simulink library "vmc"  (R2021b)
settings: Solver=VariableStepAuto  StartTime=0.0  StopTime=10.0  RelTol=1e-3
undefined symbols (not defined in the file or in its folder): AVMC_ACCDeltaTqIGain4OVRD_X_kph, AVMC_ACCDeltaTqIGain4OVRD_Y_mps2, AVMC_ACCDeltaTqIGain_X_kph, AVMC_ACCDeltaTqIGain_Y_mps2, AVMC_ACCDeltaTqPGain_X_kph, AVMC_ACCDeltaTqPGain_Y_kph, AVMC_ACCLongSteadyCtrl_X_kph, AVMC_ADSPosGFBDeltaTq_X_kph, AVMC_ADSPosGFBDeltaTq_Y_mps2, AVMC_AggressJerkPCT4AT_X_kph, AVMC_AggressJerkPCT_X_kph, AVMC_AggressLimitPCT4AT_X_kph, AVMC_AggressLimitPCT_X_kph, AVMC_CCLongSteadyCtrl_X_kph, AVMC_DISCDeltaTqIGain_X_kph, AVMC_DISCDeltaTqIGain_Y_mps2, AVMC_DISCDeltaTqPGain_X_kph, AVMC_DISCDeltaTqPGain_Y_kph, AVMC_ESCRegenOut_X_kph, AVMC_ESCRegenOut_Y_Deg, AVMC_ESCRegenOutEnSpd_X_Deg, AVMC_ISOAccLimit_X_mps, AVMC_ISODecLimit_X_mps, AVMC_ISOJerk_X_mps, AVMC_LatESCRegenOut_X_kph, AVMC_LatESCRegenOut_Y_Deg, AVMC_LongAccDeadZone_X_kph, AVMC_LongAccFiltTsforP2_X_Gps, AVMC_MCPresBaseTq_X_bar, AVMC_MSALongSteadyCtrl_X_kph, AVMC_MSAPedalOvrd_X_kph, AVMC_MSASpdBand_X_kph, AVMC_MSATqDownEndTq_X_kph, AVMC_MSATqDownTime_X_kph, AVMC_OPDDisSlideRate_X_Deg, AVMC_OVRD2ActSR2FCMCMD_X_mps2, AVMC_PedalTqRWhlRatio_X_Nm, AVMC_PedalTqRWhlRatio_Y_gps, AVMC_PedalTqRWhlSlipGain_X_rat, AVMC_PedalTqRWhlSlipGain_Y_kph, AVMC_PedalTqRWhSTRGGain_X_deg, AVMC_PedalTqRWhSTRGGain_Y_kph, AVMC_RDCDetectTime_X_kph, AVMC_RDCDetectTime_Y_pct, AVMC_RDCEnSlideRate_X_Deg, AVMC_RearWhlTqRatio_X_Nm, AVMC_RearWhlTqRatio_Y_gps, AVMC_RearWhlTqSlipGain_X_rat, AVMC_RearWhlTqSlipGain_Y_kph, AVMC_RearWhlTqSTRGGain_X_deg, AVMC_RearWhlTqSTRGGain_Y_kph, AVMC_ReqBrkJoinDecSR_X_mps2, AVMC_SoftJerkPCT_X_kph, AVMC_SoftLimitPCT_X_kph, AVMC_StESCYaw_X_kph, AVMC_StESCYaw_Y_Deg, AVMC_StESCYawCom_X_kph, AVMC_StESCYawCom_Y_Gps, AVMC_TMSpdBaseTq_X_rpm, AVMC_VehHoldDecCtrlTime2_X_kph ... (+405)
libraries: hcu_lib x105, simulink x75, tqr x1, simulink_extras x1
(part 10 of 14)

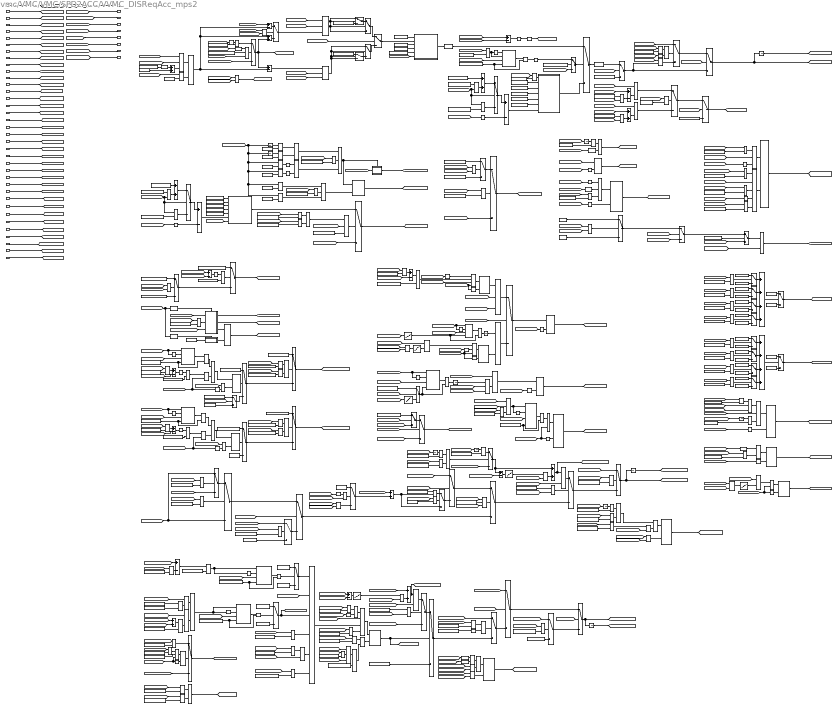
== system vmc/VMC/VMC/SPD2ACC/VVMC_DISReqAcc_mps2 ==
  note: VehHoldDelay
  note: FVT Soft Stop Control
      | (Send Hold Command after Reach H Time or ESC Standstill)
  note: Smooth Switch
      | (A, B-Pedal & REGEN to DISC)
  note: Required Acceleration for ESC
  note: Actual Required Acceleration
  note: DISC Required Acceleration
  note: Acceleration Arbitration
  note: ACC Speed Control
  note: Minimum Resolution
      | (Avoid too small command calculated from ISO Limit)
  note: Constant Speed Control
  note: ACC Constant Speed Control
  note: ACC Constant Speed Control Judgement
  VVMC_AccCalcuPID_mps2 : Inport
  VVMC_ISOJerkLimit_mps3 : Inport  Port=2
  VVMC_JerkPCT_pct : Inport  Port=3
  VVMC_ISOAccLimit_mps2 : Inport  Port=4
  VVMC_ISODecLimit_mps2 : Inport  Port=5
  VVMC_SPD2ACCAct_flg : Inport  Port=6
  VVMC_SafetyCtrl_flg : Inport  Port=7
  VINP_ACCRequiredAccel_mps2 : Inport  Port=8
  VVMC_FeatArbitrSta_enum : Inport  Port=9
  VINP_ADASACCSta_enum : Inport  Port=10
  VVMC_MeterIndSpeedForCalcu_kph : Inport  Port=11
  VVMC_FeatReqSpd_kph : Inport  Port=12
  task_time_s : Inport  Port=13
  VINP_VehSpeed_kph : Inport  Port=14
  VVMC_LongAcc_Gps : Inport  Port=15
  VVMC_LastADASWhlTqReq_Nm : Inport  Port=16
  VTQD_RrEDUAvailBrkRgnTq_Nm : Inport  Port=17
  VVMC_ACCVehHoldReqRaw_flg : Inport  Port=18
  VVMC_EstSlope_Deg : Inport  Port=19
  VTQD_FrEDUAvailBrkRgnTq_Nm : Inport  Port=20
  VVMC_ACCLowSpdTqCtrl_flg : Inport  Port=21
  VINP_GRADE_Deg : Inport  Port=22
  VINP_LFWhlRotDir_enum : Inport  Port=23
  VINP_LRWhlRotDir_enum : Inport  Port=24
  VINP_RFWhlRotDir_enum : Inport  Port=25
  VINP_RRWhlRotDir_enum : Inport  Port=26
  VVMC_ACCObjDist_m : Inport  Port=27
  VINP_MCPressure_bar : Inport  Port=28
  VDSC_PreACC_flg : Inport  Port=29
  VDSC_PreACC_mps2 : Inport  Port=30
  VDSC_DISCSta_enum : Inport  Port=31
  VDSC_AutoTurnMode_flg : Inport  Port=32
  VINP_BrkSwSta_flg : Inport  Port=33
  VINP_ACCVehHoldReq_flg : Inport  Port=34
  VTQD_GearActualPosn_enum : Inport  Port=35
  VTQD_LowIdleAccPedal_flg : Inport  Port=36
  VINP_EPBSta_enum : Inport  Port=37
  1-D Lookup Table : Lookup_n-D  NumberOfTableDimensions=1  BreakpointsForDimension1=AVMC_ReqBrkJoinDecSR_X_mps2  Table=MVMC_ReqBrkJoinDecSR_Y_mps3  InternalRulePriority=Speed  RndMeth=Simplest  InputSameDT=on
  1-D Lookup Table1 : Lookup_n-D  NumberOfTableDimensions=1  BreakpointsForDimension1=AVMC_OVRD2ActSR2FCMCMD_X_mps2  Table=MVMC_OVRD2ActSR2FCMCMD_Y_mps3  InternalRulePriority=Speed  RndMeth=Simplest  InputSameDT=on
  AND{,6,14,29} (4 alike) : Logic  Operator=OR  AllPortsSameDT=off  OutDataTypeStr=boolean
  AND{1,8,10,12,15,18..20,23..28} (14 alike) : Logic  AllPortsSameDT=off  OutDataTypeStr=boolean
  AND{3..5,11,16,21..22} (7 alike) : Logic  Inputs=3  AllPortsSameDT=off  OutDataTypeStr=boolean
  AND13 : Logic  Operator=OR  Inputs=5  AllPortsSameDT=off  OutDataTypeStr=boolean
  AND17 : Logic  Inputs=4  AllPortsSameDT=off  OutDataTypeStr=boolean
  AND2 : Logic  Inputs=4  AllPortsSameDT=off  OutDataTypeStr=boolean
  AND7 : Logic  Operator=OR  Inputs=3  AllPortsSameDT=off  OutDataTypeStr=boolean
  AND9 : Logic  Operator=OR  Inputs=3  AllPortsSameDT=off  OutDataTypeStr=boolean
  Abs{2..4,6} (4 alike) : Abs
  Add{,2,5,7,9..10,15,17..19,21,23,25} (13 alike) : Sum  Inputs=+-
  Add{1,3..4,8,11,14,16,22,24} (9 alike) : Sum
  Add12 : Sum  Inputs=++++
  Add13 : Sum  Inputs=++++
  CMDRepeat : Stateflow chart  TreatAsAtomicUnit=on
      settings: PortSchema="{\"entries\":[{\"content\":{\"sides\":[{\"content\":{\"connectorIds\":[\"In2\",\"In1\",\"In3\",\"In4\",\"In5\",\"In6\"]},\"type\":\"ConnectorPlacement.EquallySpacedRectSide\",\"uuid\":\"905b82c5-26d0-4d78-9cc9-ade9518b6cb1\"},{\"content\":{\"connectorIds\":[\"Out1\"],\"side\":\"RIGHT\"},\"type\":\"ConnectorPlacement.EquallySpacedRectSide\",\"uuid\":\"7321c4d8-dca0-41f9-ac80-faa74e816847\"},{\"content\":{\"connectorIds\":[],\"side\":\"TOP\"},\"type\":\"ConnectorPlacement.EquallySpacedRectSide\",\"uuid\":\"61a83612-f0ae-4eca-a4ee-e5180dc2049c\"}]},\"type\":\"ConnectorPlacement.EquallySpacedConnector\",\"uuid\":\"6863a8ab-8f7f-41d7-93f0-c1bbef1d5e3d\"}],\"packageUris\":[\"http://schema.mathworks.com/mf0/Connector/R2020b\"],\"version\":\"1.0\"}"
  Cast To Single : DataTypeConversion  OutDataTypeStr=single
  Cast To Single1 : DataTypeConversion  OutDataTypeStr=single
  Cast To Single7 : DataTypeConversion  OutDataTypeStr=single
  Constant : Constant  Value=pct
  Constant{1,17,27,34,38..39,42,44..45,49,64,66..68,79,81,90..92,95,108,114..115,125,127,129,131,139,141,143,145,154,163,166,175,180} (36 alike) : Constant  Value=ZERO_FLOAT
  Constant{10,94,103,107,133,147} (6 alike) : Constant  Value=TRUE
  Constant100 : Constant  Value=KVMC_VehHoldDecCtrlBSlope4ATH_mps3
  Constant101 : Constant  Value=KVMC_ReqBrkJoinWaitTime_s
  Constant{21,102,106,134,148} (5 alike) : Constant  Value=FALSE
  Constant104 : Constant  Value=KVMC_AGSVReqAccel_mps2
  Constant105 : Constant  Value=KVMC_ReqBrkJoinWaitTime_s
  Constant{7,11..12,32} (4 alike) : Constant  Value=ENUM_FEATARBITRSTA_DISC
  Constant116 : Constant  Value=KVMC_ReqBrkInDecSW_flg
  Constant{117,122..124} (4 alike) : Constant  Value=ENUM_WheelRotDir_STANDSTILL
  Constant118 : Constant  Value=KVMC_VehHoldDecCtrlBSlope_mps3
  Constant119 : Constant  Value=KVMC_VehHoldDist_m
  Constant{37,41,51,76,84,120,156,168} (8 alike) : Constant  Value=KVMC_GravityValue_mps2
  Constant{2,126,128,130,132,140,142,144,146} (9 alike) : Constant  Value=ONE_FLOAT
  Constant{6,13,33,55,61} (5 alike) : Constant  Value=ENUM_FEATARBITRSTA_ACC
  Constant{135..138} (4 alike) : Constant  Value=ENUM_WheelRotDir_BACKWARD
  Constant14 : Constant  Value=KVMC_SpdCtrlEnBand_kph
  Constant15 : Constant  Value=KVMC_VehHoldDelaySW_flg
  Constant150 : Constant  Value=KVMC_VehHoldHoldDecTime_s
  Constant151 : Constant  Value=KVMC_VehHoldDecCtrlBSlope_mps3
  Constant152 : Constant  Value=ENUM_FEATARBITRSTA_AEB
  Constant155 : Constant  Value=KVMC_VehHoldDecCtrlBSlopeCal1_mps3
  Constant157 : Constant  Value=KVMC_VehHoldHoldDecTime_s
  Constant158 : Constant  Value=KVMC_VehHoldDecCtrlBSlopeCal1_mps3
  Constant16 : Constant  Value=KVMC_Veh2MeterSpdFactor_enum
  Constant160 : Constant  Value=ENUM_VEHHOLDDELTAACCSTA_EQUAL
  Constant161 : Constant  Value=ENUM_VEHHOLDDELTAACCSTA_ACTHIGH
  Constant162 : Constant  Value=KVMC_MCPPassHoldDecTime_s
  Constant164 : Constant  Value=KVMC_VehHoldDeltaAccDB_mps2
  Constant167 : Constant  Value=KVMC_VehHoldDecCtrlBSlope_mps3
  Constant170 : Constant  Value=KVMC_VehHoldCal1BigDeltaAcc_mps2
  Constant172 : Constant  Value=KVMC_VehHoldHTimeNoMCP_bar
  Constant173 : Constant  Value=ENUM_FEATARBITRSTA_AEB
  Constant174 : Constant  Value=KVMC_VehHoldHTimeNoMCPCnt_s
  Constant176 : Constant  Value=KVMC_ReachSpeedCountTime_s
  Constant177 : Constant  Value=KVMC_ReachSpeedCount_flg
  Constant178 : Constant  Value=KVMC_DISCDecCtrlJerk_mps3
  Constant179 : Constant  Value=KVMC_DISCDecCtrlJerk_mps3
  Constant18 : Constant  Value=ENUM_ADASACCSTA_SHUTOFF
  Constant181 : Constant  Value=ENUM_DISCSTA_ACTIVE
  Constant19 : Constant  Value=ENUM_GEARACTUALPOSN_D
  Constant20 : Constant  Value=KVMC_VehHoldDecCtrlMaxDec_mps2
  Constant{22,80,85..86,99} (5 alike) : Constant  Value=ENUM_ADASACCSTA_ACTIVE
  Constant23 : Constant  Value=KVMC_Veh2MeterSpdOffset_enum
  Constant24 : Constant  Value=KVMC_SpdCtrlDisBand_kph
  Constant25 : Constant  Value=MINUSONE_FLOAT
  Constant26 : Constant  Value=KVMC_SpdCtrlReqAccel_mps2
  Constant28 : Constant  Value=KVMC_Veh2MeterSpdLoFactor_enum
  Constant29 : Constant  Value=KVMC_ADSDecShiftSW_flg
  Constant3 : Constant  Value=ZERO_INT
  Constant30 : Constant  Value=KVMC_CMDRepeatTime_enum
  Constant35 : Constant  Value=KVMC_SPD2ACCLastAccelSourceSW_flg
  Constant36 : Constant  Value=KVMC_DISCDecNoBrk_flg
  Constant4 : Constant  Value=KVMC_CMDRepeatTime_enum
  Constant40 : Constant  Value=ENUM_DISCSTA_ACTIVE
  Constant43 : Constant  Value=KVMC_AccelCtrlTqLowerLimit_Nm
  Constant46 : Constant  Value=KVMC_SprtAccelCMDSW_flg
  Constant47 : Constant  Value=KVMC_TqAccelCtrlBand_mps2
  Constant48 : Constant  Value=ENUM_EPBSTA_APPLIED
  Constant5 : Constant  Value=ENUM_FEATARBITRSTA_ACCDISC
  Constant52 : Constant  Value=KVMC_VehHoldDeltaAccDB_mps2
  Constant53 : Constant  Value=KVMC_ReqAccelLowerLimit_mps2
  Constant54 : Constant  Value=KVMC_ReqDecelLowerLimit_mps2
  Constant56 : Constant  Value=ENUM_FEATARBITRSTA_ACCDISC
  Constant57 : Constant  Value=KVMC_SpdCtrlEnBand_kph
  Constant58 : Constant  Value=KVMC_Veh2MeterSpdFactor_enum
  Constant59 : Constant  Value=KVMC_Veh2MeterSpdOffset_enum
  Constant60 : Constant  Value=KVMC_SpdCtrlDisBand_kph
  Constant62 : Constant  Value=MINUSONE_FLOAT
  Constant63 : Constant  Value=KVMC_SpdCtrlReqAccel_mps2
  Constant65 : Constant  Value=KVMC_Veh2MeterSpdLoFactor_enum
  Constant69 : Constant  Value=ENUM_VEHHOLDDELTAACCSTA_EQUAL
  Constant70 : Constant  Value=ENUM_VEHHOLDDELTAACCSTA_ACTLOW
  Constant71 : Constant  Value=KVMC_ACCSpdCtrlSW_flg
  Constant73 : Constant  Value=KVMC_ADASWhlTqLimRat_rat
  Constant74 : Constant  Value=KVMC_VehHoldDecCtrl_flg
  Constant75 : Constant  Value=KVMC_OVRD2ActRampSW_flg
  Constant77 : Constant  Value=ENUM_VEHHOLDDELTAACCSTA_EQUAL
  Constant78 : Constant  Value=ENUM_VEHHOLDDELTAACCSTA_ACTLOW
  Constant8 : Constant  Value=ENUM_FEATARBITRSTA_ACCDISC
  Constant82 : Constant  Value=KVMC_CallBrkJoinSpd_kph
  Constant83 : Constant  Value=ENUM_ADASACCSTA_OVERRIDE
  Constant87 : Constant  Value=ENUM_ADASACCSTA_OVERRIDE
  Constant88 : Constant  Value=KVMC_ADASWhlTqLimRat_rat
  Constant89 : Constant  Value=KVMC_ADSDecAlwaysShift_flg
  Constant9 : Constant  Value=KVMC_VehHoldDelayMCP_bar
  Constant93 : Constant  Value=ENUM_VEHHOLDDELTAACCSTA_ACTHIGH
  Constant96 : Constant  Value=KVMC_ADSDecRspsRatio_rat
  Constant97 : Constant  Value=KVMC_VehHoldDeltaAccDB_mps2
  ConstantSpeedControl : Stateflow chart  TreatAsAtomicUnit=on
      settings: PortSchema="{\"entries\":[{\"content\":{\"sides\":[{\"content\":{\"connectorIds\":[\"In1\",\"In3\",\"In4\",\"In5\",\"In6\",\"In7\",\"In2\"]},\"type\":\"ConnectorPlacement.EquallySpacedRectSide\",\"uuid\":\"931d4d55-b643-4b97-a7aa-1deb2b509e83\"},{\"content\":{\"connectorIds\":[\"Out1\"],\"side\":\"RIGHT\"},\"type\":\"ConnectorPlacement.EquallySpacedRectSide\",\"uuid\":\"f2f28b13-6937-4f35-b44e-683edec0d4ba\"},{\"content\":{\"connectorIds\":[],\"side\":\"TOP\"},\"type\":\"ConnectorPlacement.EquallySpacedRectSide\",\"uuid\":\"e2886b86-de2a-4a68-b05f-bfb0f2051baf\"}]},\"type\":\"ConnectorPlacement.EquallySpacedConnector\",\"uuid\":\"cece4c76-e980-42e8-adab-da09fec387c1\"}],\"packageUris\":[\"http://schema.mathworks.com/mf0/Connector/R2020b\"],\"version\":\"1.0\"}"
  ConstantSpeedControl1 : Stateflow chart  TreatAsAtomicUnit=on
      settings: PortSchema="{\"entries\":[{\"content\":{\"sides\":[{\"content\":{\"connectorIds\":[\"In2\",\"In3\",\"In4\",\"In5\",\"In6\",\"In1\",\"In7\"]},\"type\":\"ConnectorPlacement.EquallySpacedRectSide\",\"uuid\":\"931d4d55-b643-4b97-a7aa-1deb2b509e83\"},{\"content\":{\"connectorIds\":[\"Out1\"],\"side\":\"RIGHT\"},\"type\":\"ConnectorPlacement.EquallySpacedRectSide\",\"uuid\":\"f2f28b13-6937-4f35-b44e-683edec0d4ba\"},{\"content\":{\"connectorIds\":[],\"side\":\"TOP\"},\"type\":\"ConnectorPlacement.EquallySpacedRectSide\",\"uuid\":\"e2886b86-de2a-4a68-b05f-bfb0f2051baf\"}]},\"type\":\"ConnectorPlacement.EquallySpacedConnector\",\"uuid\":\"cece4c76-e980-42e8-adab-da09fec387c1\"}],\"packageUris\":[\"http://schema.mathworks.com/mf0/Connector/R2020b\"],\"version\":\"1.0\"}"
  Detect Decrease : simulink/Logic and Bit Operations/Detect Decrease  vinit=0.0  OutDataTypeStr=boolean
  Detect Increase{,1..3,5..7} (7 alike) : simulink/Logic and Bit Operations/Detect Increase  vinit=0.0  OutDataTypeStr=boolean
  Divide : Product  Inputs=*/
  Divide1 : Product  Inputs=***
  Divide{2,4..22} (20 alike) : Product  Inputs=**
  Divide24 : Product  Inputs=*/
  InitialCondition: 0 : UnitDelay  SampleTime=-1  HasFrameUpgradeWarning=on
  InitialCondition: 0 (1) : UnitDelay  SampleTime=-1  HasFrameUpgradeWarning=on
  Logical Operator2 : Logic  Operator=OR  Inputs=6  AllPortsSameDT=off  OutDataTypeStr=boolean
  Logical Operator4 : Logic  Inputs=3  AllPortsSameDT=off  OutDataTypeStr=boolean
  Logical Operator5 : Logic  Operator=OR  AllPortsSameDT=off  OutDataTypeStr=boolean
  MVMC_VehHoldDecCtrlTime2_Y : Lookup_n-D  NumberOfTableDimensions=1  BreakpointsForDimension1=AVMC_VehHoldDecCtrlTime2_X_kph  Table=MVMC_VehHoldDecCtrlTime2_Y_s  InternalRulePriority=Speed  RndMeth=Simplest  InputSameDT=on
  MVMC_VehHoldDecCtrlTime_Y_s1 : Lookup_n-D  NumberOfTableDimensions=1  BreakpointsForDimension1=AVMC_VehHoldDecCtrlTime_X_kph  Table=MVMC_VehHoldDecCtrlTime_Y_s  InternalRulePriority=Speed  RndMeth=Simplest  InputSameDT=on
  MVMC_VehHoldMCPPass2_Y_bar : Lookup_n-D  NumberOfTableDimensions=1  BreakpointsForDimension1=AVMC_VehHoldMCPPass2_X_deg  Table=MVMC_VehHoldMCPPass2_Y_bar  InternalRulePriority=Speed  RndMeth=Simplest  InputSameDT=on
  MVMC_VehHoldMCPPass_Y_bar : Lookup_n-D  NumberOfTableDimensions=1  BreakpointsForDimension1=AVMC_VehHoldMCPPass_X_deg  Table=MVMC_VehHoldMCPPass_Y_bar  InternalRulePriority=Speed  RndMeth=Simplest  InputSameDT=on
  Max1 : MinMax  Function=max  Inputs=2
  Max5 : MinMax  Function=max  Inputs=2
  Merge3 : Merge
  Min1 : MinMax  Inputs=2
  Min2 : MinMax  Function=max  Inputs=2
  Min3 : MinMax  Inputs=2
  Min4 : MinMax  Function=max  Inputs=2
  Min5 : MinMax  Inputs=2
  Min6 : MinMax  Function=max  Inputs=2
  MinMax2 : MinMax  Inputs=3
  MinMax3 : MinMax  Function=max  Inputs=3
  NOT{,1..27,29..31,33..34} (33 alike) : Logic  Operator=NOT  AllPortsSameDT=off  OutDataTypeStr=boolean
  OR{,1..4,10..15,18,20} (13 alike) : Logic  Operator=OR  AllPortsSameDT=off  OutDataTypeStr=boolean
  OR{5,16..17,21} (4 alike) : Logic  AllPortsSameDT=off  OutDataTypeStr=boolean
  OR19 : Logic  Inputs=3  AllPortsSameDT=off  OutDataTypeStr=boolean
  OR6 : Logic  Operator=OR  Inputs=3  AllPortsSameDT=off  OutDataTypeStr=boolean
  OR7 : Logic  Operator=OR  Inputs=3  AllPortsSameDT=off  OutDataTypeStr=boolean
  OR8 : Logic  Inputs=3  AllPortsSameDT=off  OutDataTypeStr=boolean
  OR9 : Logic  Operator=OR  Inputs=3  AllPortsSameDT=off  OutDataTypeStr=boolean
  Relational Operator{,1..3,5,12..14,21..23,27..28,33,43,49..56,58..59,61,69,78..79,83..86} (33 alike) : RelationalOperator  Operator===  OutDataTypeStr=boolean  RndMeth=Simplest
  Relational Operator{4,8,10,20,24..25,35,46,62} (9 alike) : RelationalOperator  Operator=<  OutDataTypeStr=boolean  RndMeth=Simplest
  Relational Operator{6,9,15..16,18,29,31,41,48,60,67..68,71,82} (14 alike) : RelationalOperator  Operator=<=  OutDataTypeStr=boolean  RndMeth=Simplest
  Relational Operator{17,19,30,32,39..40,42,57,63,65,70,72,75} (13 alike) : RelationalOperator  OutDataTypeStr=boolean  RndMeth=Simplest
  Relational Operator{26,34,36,45,47,64,66,73,76,81} (10 alike) : RelationalOperator  Operator=>  OutDataTypeStr=boolean  RndMeth=Simplest
  Relational Operator38 : RelationalOperator  Operator=~=  OutDataTypeStr=boolean  RndMeth=Simplest
  Relational Operator74 : RelationalOperator  Operator=~=  OutDataTypeStr=boolean  RndMeth=Simplest
  Relational Operator77 : RelationalOperator  Operator=~=  OutDataTypeStr=boolean  RndMeth=Simplest
  Round : Rounding  Operator=round
  Round3 : Rounding  Operator=round
  Round4 : Rounding  Operator=round
  SR_Latch{,1..17} (18 alike) : hcu_lib/Basic_Blocks/SR_Latch
  Switch : Switch  Criteria=u2 > Threshold  Threshold=KVMC_Veh2MeterSpdLoBdy_kph
  Switch1 : Switch  Criteria=u2 > Threshold  Threshold=KVMC_Veh2MeterSpdLoBdy_kph
  Switch{2..3,5..11,14,16..21,23..25,27..30,32..37,39,41..44,49} (35 alike) : Switch  Criteria=u2 > Threshold
  Switch26 : Switch  Threshold=TWO_FLOAT
  Switch31 : Switch  Threshold=TWO_FLOAT
  Timer{,1..3,5..8} (8 alike) : hcu_lib/Basic_Blocks/Timer
  Triggered Subsystem4 : Subsystem  TreatAsAtomicUnit=on
  Triggered Subsystem6 : Subsystem  TreatAsAtomicUnit=on
  Triggered Subsystem7 : Subsystem  TreatAsAtomicUnit=on
  Unit Delay{1..7,9..12} (11 alike) : UnitDelay  SampleTime=-1  HasFrameUpgradeWarning=on
  u2 > 0 (1){,1..13,15} (15 alike) : Switch  Criteria=u2 > Threshold
  u2 > 0 (10) : Switch  Criteria=u2 > Threshold
  u2 > 0 (11) : Switch  Criteria=u2 > Threshold
  u2 > 0 (16)1 : Switch  Criteria=u2 > Threshold  Threshold=KVMC_ReqAccelLowerLimit_mps2
  u2 > 0 (16)2 : Switch  Criteria=u2 > Threshold  Threshold=KVMC_ReqDecelLowerLimit_mps2
  u2 > 0 (2) : Switch  Criteria=u2 > Threshold
  u2 > 0 (5) : Switch  Criteria=u2 > Threshold
  u2 > 0 (7) : Switch  Criteria=u2 > Threshold
  u2 > 0 (9) : Switch  Criteria=u2 > Threshold
  u2 >= 0 : Switch
  "VVMC_ACCRequiredAccel_mps2 " : Outport
  VVMC_FeatArbitrFinal_enum : Outport  Port=2
  VVMC_ActACCRequiredAccel_mps2 : Outport  Port=3
  VVMC_VehHoldDecCtrlHEnd_flg : Outport  Port=4
  VVMC_DISCReqAcc_mps2 : Outport  Port=5
  VVMC_AccelTurnHold_flg : Outport  Port=6
  VVMC_ACCVehHoldReq_flg : Outport  Port=7
  VVMC_ACCShutOffHold_flg : Outport  Port=8
  VVMC_OVRD2ActRampActive_flg : Outport  Port=9
  wires:
  Switch42/1 -> InitialCondition: 0 (1)/1, [VVMC_DISCReqAcc_mps2]  "VVMC_DISCReqAcc_mps2"
  Switch2/1 -> [VVMC_JerkSource_mps2], Add/1, Add1/2  "VVMC_JerkSource_mps2"
  [VVMC_DISCReqAcc_mps2] -> u2 > 0 (9)/1, u2 > 0 (2)/3
  Relational Operator5/1 -> u2 > 0 (9)/2
  [VVMC_AfterCtrlACCReqAccel_mps2] -> u2 > 0 (9)/3
  InitialCondition: 0/1 -> [VVMC_LastActACCRequiredAccel_mps2]  "VVMC_LastActACCRequiredAccel_mps2"
  u2 > 0 (5)/1 -> u2 > 0 (1)/3
  u2 > 0 (2)/1 -> u2 > 0 (1)/1
  [VVMC_SPD2ACCAct_flg] -> u2 > 0 (1)/2
  [VVMC_FeatArbitrSta_enum] -> Relational Operator1/1
  [VVMC_FeatArbitrSta_enum] -> Relational Operator2/1
  Constant1/1 -> u2 > 0 (5)/3
  Constant11/1 -> Relational Operator5/2
  Constant5/1 -> Relational Operator1/2
  Relational Operator1/1 -> u2 > 0 (2)/2
  Constant6/1 -> Relational Operator2/2
  u2 > 0 (9)/1 -> u2 > 0 (2)/1
  Relational Operator2/1 -> u2 > 0 (5)/2
  [VVMC_AfterCtrlACCReqAccel_mps2] -> u2 > 0 (5)/1
  u2 > 0 (1)9/1 -> [VVMC_ActACCRequiredAccel_mps2], InitialCondition: 0/1  "VVMC_ActACCRequiredAccel_mps2"
  [VVMC_FeatArbitrFinal_enum] -> Relational Operator5/1
  task_time_s/1 -> [task_time_s]
  [VVMC_MeterIndSpeedForCalcu_kph] -> Add2/2
  [VVMC_FeatReqSpd_kph] -> Add2/1
  u2 > 0 (11)/1 -> Cast To Single1/1
  Abs2/1 -> Round/1
  Add2/1 -> Abs2/1
  VVMC_MeterIndSpeedForCalcu_kph/1 -> [VVMC_MeterIndSpeedForCalcu_kph]
  VVMC_FeatReqSpd_kph/1 -> [VVMC_FeatReqSpd_kph]
  Cast To Single7/1 -> u2 > 0 (11)/1  "VVMC_DISCReqAccAftRepeat_mps2"
  InitialCondition: 0 (1)/1 -> [VVMC_LastDISCReqAcc_mps2]  "VVMC_LastDISCReqAcc_mps2"
  Constant13/1 -> u2 > 0 (10)/1
  Constant12/1 -> u2 > 0 (10)/3
  Relational Operator6/1 -> u2 > 0 (10)/2
  [VVMC_AfterCtrlACCReqAccel_mps2] -> Relational Operator6/1
  [VVMC_DISCReqAcc_mps2] -> Relational Operator6/2
  VINP_ADASACCSta_enum/1 -> [VINP_ADASACCSta_enum]
  [VVMC_FeatArbitrFinal_enum] -> VVMC_FeatArbitrFinal_enum/1
  u2 > 0 (7)/1 -> [VVMC_FeatArbitrFinal_enum]  "VVMC_FeatArbitrFinal_enum"
  [VVMC_FeatArbitrSta_enum] -> u2 > 0 (7)/3
  u2 > 0 (10)/1 -> u2 > 0 (7)/1
  Relational Operator3/1 -> u2 > 0 (7)/2
  [VVMC_FeatArbitrSta_enum] -> Relational Operator3/1
  Constant8/1 -> Relational Operator3/2
  VVMC_FeatArbitrSta_enum/1 -> [VVMC_FeatArbitrSta_enum]
  VINP_ACCRequiredAccel_mps2/1 -> [VINP_ACCRequiredAccel_mps2]
  VVMC_SafetyCtrl_flg/1 -> [VVMC_SafetyCtrl_flg]
  Constant4/1 -> CMDRepeat/5(KVMC_CMDRepeatTime_enum)
  Constant3/1 -> CMDRepeat/4(ZERO_INT)
  [VVMC_ACCRequiredAccel_mps2] -> "VVMC_ACCRequiredAccel_mps2 "/1
  [VVMC_ISOJerkLimit_mps3] -> Divide1/1
  Constant/1 -> Divide/2
  VVMC_SPD2ACCAct_flg/1 -> [VVMC_SPD2ACCAct_flg]
  VVMC_ISODecLimit_mps2/1 -> [VVMC_ISODecLimit_mps2]
  VVMC_ISOAccLimit_mps2/1 -> [VVMC_ISOAccLimit_mps2]
  VVMC_JerkPCT_pct/1 -> [VVMC_JerkPCT_pct]
  VVMC_ISOJerkLimit_mps3/1 -> [VVMC_ISOJerkLimit_mps3]
  VVMC_AccCalcuPID_mps2/1 -> [VVMC_AccCalcuPID_mps2]
  [VVMC_AccCalcuPID_mps2] -> u2 >= 0/2
  [VVMC_AccCalcuPID_mps2] -> MinMax3/3
  [VVMC_AccCalcuPID_mps2] -> MinMax2/1
  [VVMC_JerkPCT_pct] -> Divide/1
  Divide1/1 -> Divide2/1
  [VVMC_ISODecLimit_mps2] -> MinMax3/2
  Divide2/1 -> Add/2, Add23/2, Add1/1  "VVMC_ISOJerkLimitFinal_mps3"
  MinMax2/1 -> Switch49/3, Switch49/2, u2 > 0 (16)1/2, u2 > 0 (16)1/1
  [VVMC_ISOAccLimit_mps2] -> MinMax2/2
  Divide/1 -> Divide2/2
  u2 >= 0/1 -> CMDRepeat/1(VVMC_DISCReqAccAftLim_mps2)  "VVMC_DISCReqAccAftLim_mps2"
  CMDRepeat/1(VVMC_DISCReqAccAftRepeat_mps2) -> Cast To Single7/1
  Add/1 -> MinMax3/1
  VINP_VehSpeed_kph/1 -> [VINP_VehSpeed_kph]
  Divide5/1 -> Add4/2
  [VINP_VehSpeed_kph] -> Switch/2, Divide8/1, Divide5/2
  Constant23/1 -> Add4/1
  Constant16/1 -> Divide5/1
  Add4/1 -> Switch/1
  Round3/1 -> Add5/2
  Add5/1 -> ConstantSpeedControl/2(DeltaSpeed)
  Constant14/1 -> ConstantSpeedControl/3(KVMC_SpdCtrlEnBand_kph)
  Constant24/1 -> ConstantSpeedControl/4(KVMC_SpdCtrlDisBand_kph)
  Constant25/1 -> ConstantSpeedControl/5(MINUSONE_FLOAT)
  [VVMC_FeatReqSpd_kph] -> Round3/1
  Constant26/1 -> ConstantSpeedControl/6(KVMC_SpdCtrlReqAccel_mps2)
  Constant27/1 -> ConstantSpeedControl/7(ZERO_FLOAT)
  Divide8/1 -> Switch/3
  Constant28/1 -> Divide8/2
  Switch/1 -> Add5/1
  ConstantSpeedControl/1(ReqAccel) -> u2 > 0 (11)/3  "VVMC_DISCConSpdCtrlCMD_mps2"
  [VVMC_SPD2ACCAct_flg] -> Detect Increase/1
  VVMC_LongAcc_Gps/1 -> [VVMC_LongAcc_Gps]
  Constant35/1 -> Logical Operator4/2
  Detect Increase/1 -> Logical Operator4/1
  Logical Operator4/1 -> Switch2/2
  [VVMC_LastDISCReqAcc_mps2] -> Switch2/3
  [VVMC_LongAcc_Gps] -> Unit Delay1/1
  Constant37/1 -> Divide9/2
  Divide9/1 -> Switch2/1
  [VVMC_SPD2ACCAct_flg] -> Switch7/2
  Constant42/1 -> Switch7/3
  Constant49/1 -> Relational Operator19/2
  Constant45/1 -> u2 > 0 (1)1/3
  Logical Operator2/1 -> AND2/3
  [VVMC_LongAcc_Gps] -> Divide10/1
  Constant47/1 -> Relational Operator18/2
  [VVMC_ActACCRequiredAccel_mps2] -> Relational Operator19/1
  Constant44/1 -> Relational Operator17/2
  Relational Operator17/1 -> AND/1
  [VVMC_LastADASWhlTqReq_Nm] -> Relational Operator15/1
  u2 > 0 (1)1/1 -> u2 > 0 (1)3/3
  Constant46/1 -> NOT/1
  NOT/1 -> AND/2
  AND/1 -> u2 > 0 (1)3/2
  Relational Operator15/1 -> Logical Operator5/2
  [VTQD_RrEDUAvailBrkRgnTq_Nm] -> Add14/1
  Relational Operator16/1 -> Logical Operator5/1
  Constant43/1 -> Divide22/1
  [VVMC_ActACCRequiredAccel_mps2] -> Relational Operator17/1
  [VVMC_ActACCReqAcc4ADS_mps2] -> u2 > 0 (1)2/1
  [VVMC_ACCVehHoldReqRaw_flg] -> u2 > 0 (1)2/2
  Add7/1 -> Relational Operator18/1
  [VVMC_ActACCRequiredAccel_mps2] -> Add7/1
  SR_Latch3/1 -> [VVMC_ReqBrkJoin_flg], u2 > 0 (1)1/2  "VVMC_ReqBrkJoin_flg"
  u2 > 0 (1)3/1 -> u2 > 0 (1)2/3
  [VVMC_LastADASWhlTqReq_Nm] -> Relational Operator16/1
  Divide10/1 -> Add7/2
  Constant41/1 -> Divide10/2
  [VVMC_ActACCRequiredAccel_mps2] -> u2 > 0 (1)3/1
  u2 > 0 (1)4/1 -> [VVMC_ACCRequiredAccel_mps2], Unit Delay6/1
  Relational Operator13/1 -> OR/1
  Constant32/1 -> Relational Operator13/2
  Constant33/1 -> Relational Operator14/2
  OR/1 -> [VVMC_ReqAccelActive_flg]  "VVMC_ReqAccelActive_flg"
  [VVMC_FeatArbitrFinal_enum] -> Relational Operator13/1
  [VVMC_FeatArbitrFinal_enum] -> Relational Operator14/1
  Relational Operator14/1 -> OR/2
  [VVMC_ReqAccelActive_flg] -> u2 > 0 (1)4/2
  u2 > 0 (1)2/1 -> u2 > 0 (1)4/1
  Constant34/1 -> u2 > 0 (1)11/3
  [VVMC_ReqAccelActive_flg] -> AND2/2
  [VVMC_ActACCRequiredAccel_mps2] -> Relational Operator20/1
  Constant39/1 -> Relational Operator20/2
  Relational Operator20/1 -> AND2/4
  VTQD_RrEDUAvailBrkRgnTq_Nm/1 -> [VTQD_RrEDUAvailBrkRgnTq_Nm]
  VVMC_LastADASWhlTqReq_Nm/1 -> [VVMC_LastADASWhlTqReq_Nm]
  [VVMC_ActACCRequiredAccel_mps2] -> VVMC_ActACCRequiredAccel_mps2/1
  Constant53/1 -> u2 > 0 (16)1/3
  u2 > 0 (16)1/1 -> Switch49/1
  Constant54/1 -> u2 > 0 (16)2/1
  MinMax3/1 -> Switch6/2, Switch6/1, u2 > 0 (16)2/2, u2 > 0 (16)2/3
  Unit Delay1/1 -> Divide9/1
  AND1/1 -> Logical Operator2/5
  Relational Operator21/1 -> AND1/1
  [VVMC_FeatArbitrFinal_enum] -> Relational Operator21/1
  Constant61/1 -> Relational Operator21/2
  [VVMC_SafetyCtrl_flg] -> AND1/2
  Constant55/1 -> Relational Operator22/2
  [VVMC_FeatArbitrSta_enum] -> Relational Operator22/1
  Constant56/1 -> Relational Operator23/2
  [VVMC_FeatArbitrSta_enum] -> Relational Operator23/1
  Relational Operator23/1 -> OR1/1
  Relational Operator22/1 -> OR1/2
  Constant58/1 -> Divide11/1
  [VINP_VehSpeed_kph] -> Switch1/2, Divide12/1, Divide11/2
  Divide11/1 -> Add8/2
  Constant65/1 -> Divide12/2
  ConstantSpeedControl1/1(ReqAccel) -> Switch5/1  "VVMC_ACCConSpdCtrlCMD_mps2"
  Add9/1 -> ConstantSpeedControl1/1(DeltaSpeed)
  Constant63/1 -> ConstantSpeedControl1/5(KVMC_SpdCtrlReqAccel_mps2)
  Constant64/1 -> ConstantSpeedControl1/6(ZERO_FLOAT)
  [VVMC_ACCReqSpdMemory_kph] -> Round4/1
  Constant60/1 -> ConstantSpeedControl1/3(KVMC_SpdCtrlDisBand_kph)
  Switch1/1 -> Add9/1
  Divide12/1 -> Switch1/3
  Constant59/1 -> Add8/1
  Add8/1 -> Switch1/1
  Constant57/1 -> ConstantSpeedControl1/2(KVMC_SpdCtrlEnBand_kph)
  Round4/1 -> Add9/2
  Constant62/1 -> ConstantSpeedControl1/4(MINUSONE_FLOAT)
  Unit Delay2/1 -> Relational Operator24/1
  Constant66/1 -> Relational Operator24/2
  OR5/1 -> AND3/3
  Relational Operator24/1 -> OR4/1
  AND3/1 -> SR_Latch4/1, Triggered Subsystem4/Trigger
  Triggered Subsystem4/1(Out1) -> [VVMC_ACCReqSpdMemory_kph]  "VVMC_ACCReqSpdMemory_kph"
  SR_Latch4/1 -> [VVMC_ACCSpdCtrl_flg]  "VVMC_ACCSpdCtrl_flg"
  OR1/1 -> AND4/1
  [VVMC_ACCSpdCtrl_flg] -> AND4/2
  Constant71/1 -> AND4/3
  AND4/1 -> Switch5/2
  [VINP_ACCRequiredAccel_mps2] -> Switch5/3
  Switch5/1 -> [VVMC_AfterCtrlACCReqAccel_mps2]  "VVMC_AfterCtrlACCReqAccel_mps2"
  VVMC_ACCVehHoldReqRaw_flg/1 -> [VVMC_ACCVehHoldReqRaw_flg]
  [VVMC_ACCVehHoldReqRaw_flg] -> AND5/1
  Constant74/1 -> AND5/2
  AND5/1 -> u2 > 0 (1)5/2
  VVMC_EstSlope_Deg/1 -> [VVMC_EstSlope_Deg]
  [VVMC_ACCVehHoldReqRaw_flg] -> Detect Decrease/1, Detect Increase2/1
  Detect Increase2/1 -> Triggered Subsystem6/Trigger
  [VVMC_LastActACCRequiredAccel_mps2] -> Triggered Subsystem6/3(In3)
  Merge3/1 -> [VVMC_VehHoldEnReqAccel_mps2]  "VVMC_VehHoldEnReqAccel_mps2"
  Constant79/1 -> Triggered Subsystem7/1(In1)
  Detect Decrease/1 -> Triggered Subsystem7/Trigger
  Triggered Subsystem6/3(Out3) -> Merge3/1
  Triggered Subsystem7/1(Out1) -> Merge3/2
  Switch33/1 -> [VVMC_VehHoldDecCtrlBSlope_mps3]  "VVMC_VehHoldDecCtrlBSlope_mps3"
  [VVMC_LastActACCRequiredAccel_mps2] -> Add11/1
  Switch9/1 -> Add11/2
  [VVMC_ACCVehHoldReqRaw_flg] -> NOT1/1, Timer/1
  NOT1/1 -> Timer/2
  [task_time_s] -> Timer/3
  MVMC_VehHoldDecCtrlTime_Y_s1/1 -> Relational Operator30/2, Timer/4
  Timer/1 -> Relational Operator30/1
  Constant81/1 -> Switch9/1
  [task_time_s] -> Divide16/2
  [VVMC_VehHoldDecCtrlBSlope_mps3] -> Divide16/1
  Divide16/1 -> Switch9/3
  [VVMC_VehHoldDecCtrlBEnd_flg] -> OR3/2
  [VVMC_ACCVehHoldReqRaw_flg] -> NOT2/1
  NOT2/1 -> OR3/1
  OR3/1 -> Switch9/2
  [VVMC_VehHoldDecCtrlBEnd_flg] -> NOT3/1, Timer1/1
  [task_time_s] -> Timer1/3
  MVMC_VehHoldDecCtrlTime2_Y/1 -> Switch21/3
  Timer1/1 -> Relational Operator32/1
  SR_Latch12/1 -> [VVMC_VehHoldDecCtrlHEnd_flg]  "VVMC_VehHoldDecCtrlHEnd_flg"
  Add11/1 -> Min1/2, Switch8/3
  [VVMC_VehHoldDecCtrlHEnd_flg] -> u2 > 0 (1)6/2
  u2 > 0 (1)6/1 -> u2 > 0 (1)5/1  "VVMC_VehHoldDecCtrlAccel_mps2"
  [VVMC_VehHoldDecCtrlHEnd_flg] -> VVMC_VehHoldDecCtrlHEnd_flg/1
  Relational Operator30/1 -> Unit Delay3/1
  [VVMC_ACCVehHoldReqRaw_flg] -> AND8/1
  Relational Operator32/1 -> Unit Delay4/1
  Unit Delay4/1 -> AND7/1
  Constant90/1 -> Relational Operator34/2
  Unit Delay5/1 -> Relational Operator34/1
  Relational Operator34/1 -> OR4/2
  Constant92/1 -> Relational Operator36/2
  Constant91/1 -> Relational Operator35/2
  Relational Operator36/1 -> NOT4/1
  NOT4/1 -> OR5/2
  Relational Operator35/1 -> NOT5/1
  NOT5/1 -> OR5/1
  OR4/1 -> AND3/1
  Constant67/1 -> Relational Operator25/2
  Constant68/1 -> Relational Operator26/2
  [VINP_ACCRequiredAccel_mps2] -> Unit Delay2/1, Relational Operator36/1, Relational Operator26/1, Relational Operator25/1, Relational Operator35/1, Unit Delay5/1
  Relational Operator25/1 -> OR6/1
  Relational Operator26/1 -> OR6/3
  AND7/1 -> AND8/2
  VTQD_FrEDUAvailBrkRgnTq_Nm/1 -> [VTQD_FrEDUAvailBrkRgnTq_Nm]
  [VTQD_FrEDUAvailBrkRgnTq_Nm] -> Add14/2
  NOT3/1 -> Timer1/2
  VVMC_ACCLowSpdTqCtrl_flg/1 -> [VVMC_ACCLowSpdTqCtrl_flg]
  [VVMC_ACCLowSpdTqCtrl_flg] -> Logical Operator2/2
  [VINP_VehSpeed_kph] -> Relational Operator31/1
  Constant82/1 -> Relational Operator31/2
  Relational Operator31/1 -> Logical Operator2/4
  [VVMC_SPD2ACCAct_flg] -> CMDRepeat/6(VVMC_SPD2ACCAct_flg)
  Constant94/1 -> CMDRepeat/2(TRUE)
  Constant95/1 -> CMDRepeat/3(ZERO_FLOAT)
  [VVMC_MeterIndSpeedForCalcu_kph] -> Triggered Subsystem4/1(In1)
  Relational Operator38/1 -> OR6/2
  Constant101/1 -> Relational Operator40/2, Timer2/4
  [task_time_s] -> Timer2/3
  Logical Operator5/1 -> Timer2/1, NOT6/1
  NOT6/1 -> Timer2/2
  Timer2/1 -> Relational Operator40/1
  Relational Operator40/1 -> u2 > 0 (1)7/2
  Constant102/1 -> u2 > 0 (1)7/3
  u2 > 0 (1)7/1 -> [VVMC_ADASWhlTqReachLim_flg], Logical Operator2/3  "VVMC_ADASWhlTqReachLim_flg"
  Constant103/1 -> u2 > 0 (1)7/1
  [VVMC_ActACCRequiredAccel_mps2] -> Relational Operator41/1
  Relational Operator41/1 -> Logical Operator2/6
  Constant104/1 -> Relational Operator41/2
  Constant107/1 -> u2 > 0 (1)8/1
  Constant106/1 -> u2 > 0 (1)8/3
  Relational Operator42/1 -> u2 > 0 (1)8/2
  Timer3/1 -> Relational Operator42/1
  NOT7/1 -> Timer3/2
  Relational Operator18/1 -> NOT7/1, Timer3/1
  [task_time_s] -> Timer3/3
  Constant105/1 -> Timer3/4, Relational Operator42/2
  u2 > 0 (1)8/1 -> Logical Operator2/1
  [VINP_VehSpeed_kph] -> Triggered Subsystem6/1(In1)
  Triggered Subsystem6/1(Out1) -> [VVMC_VehHoldEnSpd_kph]  "VVMC_VehHoldEnSpd_kph"
  [VVMC_LastActACCRequiredAccel_mps2] -> u2 > 0 (1)6/1
  [VVMC_VehHoldEnSpd_kph] -> MVMC_VehHoldDecCtrlTime_Y_s1/1
  [VVMC_VehHoldEnSpd_kph] -> MVMC_VehHoldDecCtrlTime2_Y/1
  [VVMC_ACCVehHoldReqRaw_flg] -> OR8/2
  [VVMC_ACCVehHoldReqRaw_flg] -> NOT8/1
  SR_Latch5/1 -> [VVMC_ZeroSpdHoldAllow_flg]  "VVMC_ZeroSpdHoldAllow_flg"
  [VVMC_ZeroSpdHoldAllow_flg] -> AND7/2
  VINP_GRADE_Deg/1 -> [VINP_GRADE_Deg]
  OR8/1 -> SR_Latch5/1
  VINP_LFWhlRotDir_enum/1 -> [VINP_LFWhlRotDir_enum]
  VINP_LRWhlRotDir_enum/1 -> [VINP_LRWhlRotDir_enum]
  VINP_RFWhlRotDir_enum/1 -> [VINP_RFWhlRotDir_enum]
  VINP_RRWhlRotDir_enum/1 -> [VINP_RRWhlRotDir_enum]
  [VINP_LFWhlRotDir_enum] -> Relational Operator49/1
  Constant117/1 -> Relational Operator49/2
  Constant122/1 -> Relational Operator50/2
  [VINP_LRWhlRotDir_enum] -> Relational Operator50/1
  Constant123/1 -> Relational Operator51/2
  [VINP_RFWhlRotDir_enum] -> Relational Operator51/1
  [VINP_RRWhlRotDir_enum] -> Relational Operator52/1
  Constant124/1 -> Relational Operator52/2
  Relational Operator49/1 -> Switch14/2
  Constant125/1 -> Switch14/3
  Constant126/1 -> Switch14/1
  Constant128/1 -> Switch23/1
  Constant127/1 -> Switch23/3
  Relational Operator50/1 -> Switch23/2
  Relational Operator51/1 -> Switch24/2
  Constant129/1 -> Switch24/3
  Constant130/1 -> Switch24/1
  Constant132/1 -> Switch25/1
  Constant131/1 -> Switch25/3
  Relational Operator52/1 -> Switch25/2
  Switch25/1 -> Add12/4
  Switch24/1 -> Add12/3
  Switch23/1 -> Add12/2
  Switch14/1 -> Add12/1
  Add12/1 -> Switch26/2
  Constant133/1 -> Switch26/1
  Constant134/1 -> Switch26/3
  Switch26/1 -> [VVMC_WhlStandstill_flg]  "VVMC_WhlStandstill_flg"
  Switch31/1 -> [VVMC_WhlBackward_flg]  "VVMC_WhlBackward_flg"
  Constant148/1 -> Switch31/3
  Constant147/1 -> Switch31/1
  Add13/1 -> Switch31/2
  Switch27/1 -> Add13/1
  Switch28/1 -> Add13/2
  Switch29/1 -> Add13/3
  Switch30/1 -> Add13/4
  Relational Operator56/1 -> Switch30/2
  Constant145/1 -> Switch30/3
  Constant146/1 -> Switch30/1
  Constant144/1 -> Switch29/1
  Constant143/1 -> Switch29/3
  Relational Operator55/1 -> Switch29/2
  Relational Operator54/1 -> Switch28/2
  Constant141/1 -> Switch28/3
  Constant142/1 -> Switch28/1
  Constant140/1 -> Switch27/1
  Constant139/1 -> Switch27/3
  Relational Operator53/1 -> Switch27/2
  Constant138/1 -> Relational Operator56/2
  [VINP_RRWhlRotDir_enum] -> Relational Operator56/1
  [VINP_RFWhlRotDir_enum] -> Relational Operator55/1
  Constant137/1 -> Relational Operator55/2
  [VINP_LRWhlRotDir_enum] -> Relational Operator54/1
  Constant136/1 -> Relational Operator54/2
  Constant135/1 -> Relational Operator53/2
  [VINP_LFWhlRotDir_enum] -> Relational Operator53/1
  OR7/1 -> OR8/1
  [VVMC_WhlStandstill_flg] -> OR7/2
  [VVMC_WhlBackward_flg] -> OR7/3
  VVMC_ACCObjDist_m/1 -> [VVMC_ACCObjDist_m]
  [VVMC_ACCObjDist_m] -> Relational Operator48/1
  Relational Operator48/1 -> OR7/1
  Constant119/1 -> Relational Operator48/2
  [VVMC_VehHoldDecCtrlBSlopeCal1_mps3] -> Switch33/3
  Switch18/1 -> Switch33/1
  Relational Operator57/1 -> AND15/1
  VINP_MCPressure_bar/1 -> [VINP_MCPressure_bar]
  [VINP_MCPressure_bar] -> Relational Operator57/1
  SR_Latch2/1 -> [VVMC_VehHoldMCPPass_flg]  "VVMC_VehHoldMCPPass_flg"
  [VINP_GRADE_Deg] -> Max5/1
  [VVMC_EstSlope_Deg] -> Max5/2
  Max5/1 -> MVMC_VehHoldMCPPass_Y_bar/1
  MVMC_VehHoldMCPPass_Y_bar/1 -> Relational Operator57/2
  [VVMC_VehHoldDecCtrlCalSW2_flg] -> Switch33/2
  AND18/1 -> SR_Latch1/1
  Detect Increase5/1 -> AND18/1
  [VVMC_ACCVehHoldReqRaw_flg] -> NOT12/1
  [VVMC_ACCVehHoldReqRaw_flg] -> Detect Increase5/1
  SR_Latch1/1 -> [VVMC_VehHoldDecCtrlCalSW2_flg]  "VVMC_VehHoldDecCtrlCalSW2_flg"
  [VVMC_ACCVehHoldReqRaw_flg] -> AND15/2, NOT10/1
  Constant152/1 -> Relational Operator59/2
  [VVMC_FeatArbitrSta_enum] -> Relational Operator59/1
  Relational Operator59/1 -> u2 > 0 (1)9/2
  [VINP_ACCRequiredAccel_mps2] -> u2 > 0 (1)9/1
  [VVMC_VehHoldDecCtrlCalSW2_flg] -> Switch21/2
  Switch21/1 -> Relational Operator32/2, Timer1/4
  Constant162/1 -> Switch21/1
  [VVMC_ActACCRequiredAccel_mps2] -> Unit Delay9/1
  Relational Operator62/1 -> OR8/3
  Constant163/1 -> Relational Operator62/2
  Unit Delay9/1 -> Relational Operator62/1
  Constant86/1 -> Relational Operator33/2
  [VINP_ADASACCSta_enum] -> Relational Operator33/1
  Relational Operator33/1 -> AND3/2
  [VINP_ADASACCSta_enum] -> Relational Operator38/1
  Constant99/1 -> Relational Operator38/2
  [VVMC_AccelTurnHold_flg] -> Switch18/2
  [VVMC_VehHoldDecCtrlBSlopeCal2_mps3] -> Switch18/3
  Constant100/1 -> Switch18/1
  [VVMC_HoldDelayAllow_flg] -> AND5/3
  [VVMC_DISCReqAcc_mps2] -> VVMC_DISCReqAcc_mps2/1
  [VVMC_ACCSpdCtrl_flg] -> NOT13/1
  NOT13/1 -> AND6/2
  [VINP_MCPressure_bar] -> Relational Operator4/1
  Constant9/1 -> Relational Operator4/2
  Relational Operator4/1 -> AND18/2
  Constant20/1 -> Min1/1
  [VINP_MCPressure_bar] -> Relational Operator8/1
  MVMC_VehHoldMCPPass2_Y_bar/1 -> Relational Operator8/2
  Relational Operator8/1 -> AND16/1
  [VVMC_ACCVehHoldReqRaw_flg] -> AND16/3, NOT17/1
  AND16/1 -> SR_Latch/1
  NOT17/1 -> SR_Latch/2
  [VVMC_VehHoldDecCtrlCalSW2_flg] -> NOT18/1
  NOT18/1 -> AND16/2
  Min1/1 -> Switch8/1
  Max1/1 -> MVMC_VehHoldMCPPass2_Y_bar/1
  [VVMC_EstSlope_Deg] -> Max1/2
  [VINP_GRADE_Deg] -> Max1/1
  [VVMC_LastACCRequiredAccel_mps2] -> Add3/1
  1-D Lookup Table/1 -> Divide15/1
  [task_time_s] -> Divide15/2
  Divide15/1 -> Add3/2
  Min2/1 -> u2 > 0 (1)10/1
  Add3/1 -> [VVMC_ACCReqAccelAfterSR_mps2], Min2/1
  u2 > 0 (1)10/1 -> u2 > 0 (1)1/1
  Constant116/1 -> AND20/1
  [VVMC_ActACCReqAcc4ADS_mps2] -> u2 > 0 (1)10/3
  NOT8/1 -> SR_Latch5/2
  NOT12/1 -> SR_Latch1/2
  NOT10/1 -> SR_Latch2/2
  AND15/1 -> SR_Latch2/1
  Relational Operator19/1 -> OR18/1
  AND2/1 -> SR_Latch3/1
  OR6/1 -> SR_Latch4/2
  [VVMC_LongAcc_Gps] -> Divide17/1
  Triggered Subsystem6/2(Out2) -> [VVMC_VehHoldEnActAccel_mps2]  "VVMC_VehHoldEnActAccel_mps2"
  Constant51/1 -> Divide17/2
  Divide17/1 -> Triggered Subsystem6/2(In2)
  [VVMC_VehHoldEnActAccel_mps2] -> Add15/1
  [VVMC_VehHoldEnReqAccel_mps2] -> Add15/2
  Add15/1 -> Abs6/1
  Abs6/1 -> Relational Operator9/1
  Constant52/1 -> Relational Operator9/2
  Relational Operator9/1 -> Switch20/2
  [VVMC_VehHoldEnActAccel_mps2] -> Relational Operator10/1
  [VVMC_VehHoldEnReqAccel_mps2] -> Relational Operator10/2
  Switch32/1 -> Switch20/3
  Relational Operator10/1 -> Switch32/2
  Constant69/1 -> Switch20/1
  Constant70/1 -> Switch32/1
  Constant93/1 -> Switch32/3
  Switch20/1 -> [VVMC_VehHoldDeltaAccSta_enum]  "VVMC_VehHoldDeltaAccSta_enum"
  Switch8/1 -> u2 > 0 (1)6/3
  Constant77/1 -> Relational Operator27/2
  [VVMC_VehHoldDeltaAccSta_enum] -> Relational Operator27/1
  [VVMC_VehHoldDeltaAccSta_enum] -> Relational Operator28/1
  Constant78/1 -> Relational Operator28/2
  Relational Operator28/1 -> OR10/2
  Relational Operator27/1 -> OR10/1
  OR10/1 -> Switch19/2
  Constant151/1 -> Switch19/1
  Switch19/1 -> [VVMC_VehHoldDecCtrlBSlopeCal2_mps3]  "VVMC_VehHoldDecCtrlBSlopeCal2_mps3"
  Switch35/1 -> Switch19/3
  Add17/1 -> Abs3/1
  Divide13/1 -> Add17/1
  [VVMC_LastActACCRequiredAccel_mps2] -> Add17/2
  Constant97/1 -> Relational Operator29/2
  Abs3/1 -> Relational Operator29/1
  Relational Operator29/1 -> OR16/1
  Switch39/1 -> Switch35/3
  SR_Latch6/1 -> Switch35/2
  Constant118/1 -> Switch35/1
  [VVMC_LongAcc_Gps] -> Divide13/1
  Constant120/1 -> Divide13/2
  [VVMC_VehHoldDecCtrlBEnd_flg] -> OR12/1
  OR11/1 -> SR_Latch6/1
  Timer5/1 -> Relational Operator39/1
  [task_time_s] -> Timer5/3
  NOT9/1 -> Timer5/2
  [VVMC_ACCVehHoldReqRaw_flg] -> NOT9/1, Timer5/1
  Constant150/1 -> Timer5/4, Relational Operator39/2
  Relational Operator39/1 -> OR11/1
  [VVMC_ACCVehHoldReqRaw_flg] -> OR16/2, NOT19/1
  NOT19/1 -> OR12/2
  OR12/1 -> SR_Latch6/2
  OR15/1 -> SR_Latch7/2
  NOT21/1 -> OR15/2
  [VVMC_ACCVehHoldReqRaw_flg] -> OR21/2, NOT21/1
  Relational Operator63/1 -> OR14/1
  Constant157/1 -> Relational Operator63/2, Timer6/4
  [VVMC_ACCVehHoldReqRaw_flg] -> Timer6/1, NOT23/1
  NOT23/1 -> Timer6/2
  [task_time_s] -> Timer6/3
  Timer6/1 -> Relational Operator63/1
  OR14/1 -> SR_Latch7/1
  [VVMC_VehHoldDecCtrlBEnd_flg] -> OR15/1
  Constant156/1 -> Divide18/2
  [VVMC_LongAcc_Gps] -> Divide18/1
  Constant155/1 -> Switch37/1
  SR_Latch7/1 -> Switch37/2
  Constant154/1 -> Switch37/3
  Relational Operator60/1 -> OR21/1
  Abs4/1 -> Relational Operator60/1
  Constant164/1 -> Relational Operator60/2
  [VVMC_LastActACCRequiredAccel_mps2] -> Add18/2
  Divide18/1 -> Add18/1
  Add18/1 -> Abs4/1
  Switch37/1 -> Switch36/3
  Switch36/1 -> [VVMC_VehHoldDecCtrlBSlopeCal1_mps3]  "VVMC_VehHoldDecCtrlBSlopeCal1_mps3"
  Constant158/1 -> Switch36/1
  OR13/1 -> Switch36/2
  Relational Operator43/1 -> OR13/1
  Relational Operator58/1 -> OR13/2
  Constant161/1 -> Relational Operator58/2
  [VVMC_VehHoldDeltaAccSta_enum] -> Relational Operator58/1
  [VVMC_VehHoldDeltaAccSta_enum] -> Relational Operator43/1
  Constant160/1 -> Relational Operator43/2
  [VVMC_VehHoldDecCtrlBSlope_mps3] -> Relational Operator64/1
  Constant166/1 -> Relational Operator64/2
  Relational Operator64/1 -> Switch8/2
  [VVMC_AccelTurnHold_flg] -> Switch39/2
  Constant167/1 -> Switch39/1
  Constant108/1 -> Switch39/3
  Relational Operator65/1 -> AND17/2
  [VVMC_LastActACCRequiredAccel_mps2] -> Add21/2
  [VVMC_ZeroSpdHoldAllow_flg] -> AND9/2
  SR_Latch8/1 -> AND9/1
  SR_Latch17/1 -> [VVMC_VehHoldDecCtrlBEnd_flg]  "VVMC_VehHoldDecCtrlBEnd_flg"
  [VVMC_VehHoldMCPPass_flg] -> AND9/3
  Unit Delay3/1 -> AND14/1
  SR_Latch/1 -> AND14/2
  AND9/1 -> Switch34/1
  AND14/1 -> Switch34/3
  NOT24/1 -> SR_Latch8/2
  Add21/1 -> Relational Operator65/1
  AND17/1 -> SR_Latch8/1
  [VVMC_ACCVehHoldReqRaw_flg] -> AND17/4, NOT24/1
  [VVMC_VehHoldDecCtrlCalSW2_flg] -> Switch34/2
  Constant170/1 -> Relational Operator65/2
  Divide21/1 -> Add21/1
  Constant168/1 -> Divide21/2
  [VVMC_LongAcc_Gps] -> Divide21/1
  [VVMC_VehHoldDecCtrlCalSW2_flg] -> AND17/3
  [VVMC_AccelTurnHold_flg] -> NOT25/1
  NOT25/1 -> AND17/1
  Unit Delay6/1 -> [VVMC_LastACCRequiredAccel_mps2]
  [VVMC_ActACCReqAcc4ADS_mps2] -> Add19/2
  [VVMC_LastACCRequiredAccel_mps2] -> Add19/1
  Add19/1 -> 1-D Lookup Table/1
  [VVMC_ReqBrkJoin_flg] -> Detect Increase3/1
  [VVMC_LastACCRequiredAccel_mps2] -> Relational Operator66/1
  [VVMC_ActACCReqAcc4ADS_mps2] -> Relational Operator66/2
  Detect Increase3/1 -> AND29/2
  Relational Operator66/1 -> AND19/2
  AND19/1 -> SR_Latch9/1
  [VVMC_ACCReqAccelAfterSR_mps2] -> Relational Operator67/1
  [VVMC_ActACCReqAcc4ADS_mps2] -> Relational Operator67/2
  Relational Operator67/1 -> SR_Latch9/2
  SR_Latch9/1 -> [VVMC_ReqBrkJoinSRActive_flg]  "VVMC_ReqBrkJoinSRActive_flg"
  [VVMC_ReqBrkJoinSRActive_flg] -> AND20/2
  AND20/1 -> u2 > 0 (1)10/2
  Cast To Single1/1 -> Switch7/1
  u2 > 0 (1)11/1 -> u2 > 0 (1)4/3
  Constant173/1 -> Relational Operator69/2
  [VVMC_FeatArbitrSta_enum] -> Relational Operator69/1
  Relational Operator69/1 -> u2 > 0 (1)11/2
  [VVMC_ActACCReqAcc4ADS_mps2] -> u2 > 0 (1)11/1
  [VVMC_VehHoldDecCtrlBEnd_flg] -> AND21/2
  [VINP_MCPressure_bar] -> Relational Operator68/1
  Constant172/1 -> Relational Operator68/2
  Relational Operator68/1 -> AND21/3
  AND21/1 -> NOT26/1, Timer7/1
  NOT26/1 -> Timer7/2
  [task_time_s] -> Timer7/3
  Constant174/1 -> Relational Operator70/2, Timer7/4
  Timer7/1 -> Relational Operator70/1
  SR_Latch15/1 -> [VVMC_VehHoldHTimeNoMCPDet_flg]  "VVMC_VehHoldHTimeNoMCPDet_flg"
  [VVMC_VehHoldDecCtrlCalSW2_flg] -> AND21/1
  [VVMC_VehHoldHTimeNoMCPDet_flg] -> AND7/3
  [VVMC_ACCSpdCtrl_flg] -> ConstantSpeedControl1/7(VVMC_ACCSpdCtrl_flg)
  [VVMC_AbsDeltaSpd_kph] -> Relational Operator71/1
  Constant175/1 -> Relational Operator71/2
  Relational Operator71/1 -> ConstantSpeedControl/1(ZeroDeltaSpd)
  u2 > 0 (1)5/1 -> u2 > 0 (1)12/3
  u2 > 0 (1)/1 -> u2 > 0 (1)5/3
  Switch6/1 -> u2 >= 0/3
  u2 > 0 (16)2/1 -> Switch6/3
  Switch49/1 -> u2 >= 0/1
  [task_time_s] -> Divide1/2
  Constant30/1 -> Cast To Single/1
  Add22/1 -> Divide1/3
  Cast To Single/1 -> Add22/1
  Constant2/1 -> Add22/2
  [VVMC_MeterIndSpeedForCalcu_kph] -> Relational Operator45/2
  [VVMC_FeatReqSpd_kph] -> Relational Operator45/1
  Relational Operator45/1 -> [VVMC_AccAct_flg]  "VVMC_AccAct_flg"
  [VVMC_AccAct_flg] -> Logical Operator4/3
  Relational Operator47/1 -> Switch17/2
  [VVMC_ISOAccLimit_mps2] -> Relational Operator47/2
  [VVMC_JerkSource_mps2] -> Relational Operator47/1
  Add1/1 -> Switch17/3
  Add23/1 -> Switch17/1
  [VVMC_JerkSource_mps2] -> Add23/1
  Switch17/1 -> MinMax2/3
  Constant176/1 -> Relational Operator72/2, Timer8/4
  Relational Operator73/1 -> Timer8/2, NOT31/1
  [task_time_s] -> Timer8/3
  Timer8/1 -> Relational Operator72/1
  Round/1 -> [VVMC_AbsDeltaSpd_kph]
  Relational Operator72/1 -> NOT30/1
  NOT30/1 -> Switch41/1  "VVMC_AbsDeltaSpdNotZero_flg"
  Constant115/1 -> Relational Operator73/2
  NOT31/1 -> Timer8/1
  Constant177/1 -> Switch41/2
  Switch41/1 -> u2 > 0 (11)/2
  [VVMC_AbsDeltaSpd_kph] -> Relational Operator73/1
  [VVMC_AbsDeltaSpd_kph] -> Switch41/3
  Relational Operator46/1 -> Switch16/2
  [VVMC_LastDISCReqAcc_mps2] -> Add24/1
  Add24/1 -> Min3/2
  Constant180/1 -> Switch43/3
  [VDSC_PreACC_flg] -> Switch43/2
  [VDSC_PreACC_mps2] -> Relational Operator46/1
  Constant114/1 -> Relational Operator46/2
  Divide19/1 -> Add24/2
  [VVMC_LastDISCReqAcc_mps2] -> Add25/1
  Switch43/1 -> [VVMC_PreACCReqAcc_mps2]  "VVMC_PreACCReqAcc_mps2"
  Divide20/1 -> Add25/2
  Constant178/1 -> Divide19/1
  [task_time_s] -> Divide19/2
  [task_time_s] -> Divide20/2
  Min4/1 -> Switch16/1
  [VDSC_PreACC_mps2] -> Min4/1
  Add25/1 -> Min4/2
  Switch16/1 -> Switch43/1
  Min3/1 -> Switch16/3
  [VDSC_PreACC_mps2] -> Min3/1
  Constant179/1 -> Divide20/1
  Min5/1 -> Switch44/3
  [VVMC_PreACCReqAcc_mps2] -> Min5/1
  [VVMC_PreACCReqAcc_mps2] -> Switch44/1
  NOT29/1 -> OR17/2
  Constant181/1 -> Relational Operator74/2
  Switch44/1 -> Switch42/1
  OR17/1 -> Switch44/2
  Relational Operator74/1 -> OR17/1
  [VDSC_PreACC_flg] -> Switch42/2
  [VDSC_DISCSta_enum] -> Relational Operator74/1
  [VDSC_AutoTurnMode_flg] -> NOT29/1
  Switch7/1 -> Min5/2, Switch42/3
  VDSC_AutoTurnMode_flg/1 -> [VDSC_AutoTurnMode_flg]
  VDSC_DISCSta_enum/1 -> [VDSC_DISCSta_enum]
  VDSC_PreACC_flg/1 -> [VDSC_PreACC_flg]
  VDSC_PreACC_mps2/1 -> [VDSC_PreACC_mps2]
  [VVMC_FeatArbitrFinal_enum] -> Relational Operator61/1
  Constant7/1 -> Relational Operator61/2
  Relational Operator61/1 -> AND6/1
  AND6/1 -> AND2/1
  Constant22/1 -> Relational Operator78/2
  AND12/1 -> [VVMC_AccelTurnHoldDet_flg]  "VVMC_AccelTurnHoldDet_flg"
  NOT22/1 -> AND13/4
  [VVMC_ACCVehHoldReqRaw_flg] -> NOT14/1
  Switch3/1 -> Switch11/1
  Constant18/1 -> Relational Operator/2
  [VVMC_ACCVehHoldReqRaw_flg] -> Detect Increase1/1
  Relational Operator79/1 -> AND13/5
  Constant15/1 -> Switch10/2
  [VVMC_ACCShutOffHold_flg] -> OR2/2
  Relational Operator78/1 -> AND13/3
  AND11/1 -> SR_Latch11/1
  NOT16/1 -> AND22/1
  SR_Latch11/1 -> [VVMC_ACCShutOffHold_flg]  "VVMC_ACCShutOffHold_flg"
  Relational Operator76/1 -> AND22/3
  AND10/1 -> Switch3/2
  Constant48/1 -> Relational Operator79/2
  AND13/1 -> SR_Latch11/2
  [VINP_ADASACCSta_enum] -> Relational Operator78/1
  [VINP_BrkSwSta_flg] -> AND13/2
  Constant19/1 -> Relational Operator77/2
  [VINP_BrkSwSta_flg] -> NOT16/1
  [VTQD_GearActualPosn_enum] -> Relational Operator77/1
  [VINP_ADASACCSta_enum] -> Relational Operator/1
  NOT15/1 -> SR_Latch13/2
  Detect Increase1/1 -> AND12/2
  Detect Increase6/1 -> AND22/2
  AND22/1 -> SR_Latch10/1
  [VVMC_ACCVehHoldReqRaw_flg] -> AND10/2
  [VVMC_ACCRequiredAccel_mps2] -> Unit Delay7/1
  Relational Operator75/1 -> AND12/1
  [VTQD_LowIdleAccPedal_flg] -> NOT22/1
  [VVMC_ACCVehHoldReqRaw_flg] -> Switch11/3
  NOT20/1 -> AND11/3
  Relational Operator77/1 -> AND13/1
  Constant21/1 -> Switch3/3
  Unit Delay7/1 -> Relational Operator75/1
  Constant38/1 -> Relational Operator75/2
  [VINP_VehSpeed_kph] -> Relational Operator76/1
  [VINP_ACCVehHoldReq_flg] -> AND11/2
  SR_Latch13/1 -> [VVMC_AccelTurnHold_flg]  "VVMC_AccelTurnHold_flg"
  [VVMC_ACCVehHoldReqRaw_flg] -> NOT15/1
  [VVMC_AccelTurnHoldDet_flg] -> SR_Latch13/1
  SR_Latch10/1 -> [VVMC_HoldDelayAllow_flg]  "VVMC_HoldDelayAllow_flg"
  [VVMC_HoldDelayAllow_flg] -> Switch11/2
  Relational Operator/1 -> AND11/1
  OR2/1 -> [VVMC_ACCVehHoldReq_flg]  "VVMC_ACCVehHoldReq_flg"
  [VVMC_VehHoldDecCtrlHEnd_flg] -> AND10/1
  [VINP_EPBSta_enum] -> Relational Operator79/1
  Constant10/1 -> Switch3/1
  [VVMC_ACCVehHoldReqRaw_flg] -> Detect Increase6/1
  Switch10/1 -> OR2/1
  [VVMC_ACCVehHoldReqRaw_flg] -> Switch10/3
  NOT14/1 -> SR_Latch10/2
  [VINP_BrkSwSta_flg] -> NOT20/1
  Switch11/1 -> Switch10/1
  Constant17/1 -> Relational Operator76/2
  VINP_BrkSwSta_flg/1 -> [VINP_BrkSwSta_flg]
  VINP_ACCVehHoldReq_flg/1 -> [VINP_ACCVehHoldReq_flg]
  VTQD_GearActualPosn_enum/1 -> [VTQD_GearActualPosn_enum]
  VTQD_LowIdleAccPedal_flg/1 -> [VTQD_LowIdleAccPedal_flg]
  VINP_EPBSta_enum/1 -> [VINP_EPBSta_enum]
  [VVMC_AccelTurnHold_flg] -> VVMC_AccelTurnHold_flg/1
  [VVMC_ACCVehHoldReq_flg] -> VVMC_ACCVehHoldReq_flg/1
  [VVMC_ACCShutOffHold_flg] -> VVMC_ACCShutOffHold_flg/1
  Constant40/1 -> Relational Operator12/2
  [VDSC_AutoTurnMode_flg] -> OR9/3
  [VDSC_PreACC_flg] -> OR9/1
  OR9/1 -> AND23/1
  Relational Operator12/1 -> OR9/2
  [VDSC_DISCSta_enum] -> Relational Operator12/1
  Constant36/1 -> AND23/2
  OR18/1 -> SR_Latch3/2
  AND23/1 -> OR18/2
  Unit Delay12/1 -> Relational Operator86/1
  [VINP_ADASACCSta_enum] -> Relational Operator85/1
  Relational Operator85/1 -> AND28/2
  Constant85/1 -> Relational Operator85/2
  [VVMC_LongAcc_Gps] -> Divide7/1
  Constant87/1 -> Relational Operator86/2
  Unit Delay10/1 -> Divide6/1
  Constant84/1 -> Divide7/2
  [VINP_ADASACCSta_enum] -> Unit Delay12/1
  Relational Operator84/1 -> AND27/1
  [VINP_ADASACCSta_enum] -> Relational Operator83/1
  Relational Operator86/1 -> AND28/1
  Unit Delay11/1 -> Relational Operator84/1
  Relational Operator83/1 -> AND27/2
  Constant76/1 -> Divide6/2
  Constant80/1 -> Relational Operator83/2
  [VINP_ADASACCSta_enum] -> Unit Delay11/1
  [VVMC_AfterCtrlACCReqAccel_mps2] -> Add10/2
  [VVMC_OVRD2ActReqAccelAftSR_mps2] -> Relational Operator82/1
  [VVMC_OVRD2ActRampActive_flg] -> AND25/2
  SR_Latch14/1 -> [VVMC_OVRD2ActRampActive_flg]  "VVMC_OVRD2ActRampActive_flg"
  [task_time_s] -> Divide4/2
  Relational Operator81/1 -> AND26/2
  [VVMC_AfterCtrlACCReqAccel_mps2] -> Relational Operator81/2
  Constant83/1 -> Relational Operator84/2
  AND27/1 -> AND26/1
  [VVMC_AfterCtrlACCReqAccel_mps2] -> Relational Operator82/2
  Min6/1 -> u2 > 0 (1)12/1
  Divide7/1 -> Relational Operator81/1
  [VVMC_AfterCtrlACCReqAccel_mps2] -> Min6/2
  Add10/1 -> 1-D Lookup Table1/1
  Add16/1 -> [VVMC_OVRD2ActReqAccelAftSR_mps2], Min6/1  "VVMC_OVRD2ActReqAccelAftSR_mps2"
  AND28/1 -> u2 > 0 (1)13/2
  AND25/1 -> u2 > 0 (1)12/2
  1-D Lookup Table1/1 -> Divide4/1
  Divide6/1 -> u2 > 0 (1)13/1
  AND26/1 -> SR_Latch14/1
  [VVMC_LongAcc_Gps] -> Unit Delay10/1
  Constant75/1 -> AND25/1
  Divide4/1 -> Add16/2
  u2 > 0 (1)13/1 -> Add10/1, Add16/1
  [VVMC_LastActACCRequiredAccel_mps2] -> u2 > 0 (1)13/3
  u2 > 0 (1)12/1 -> u2 > 0 (1)9/3
  [VVMC_ACCVehHoldReqRaw_flg] -> AND24/2, NOT33/1
  AND24/1 -> SR_Latch15/1
  Relational Operator70/1 -> AND24/1
  NOT33/1 -> SR_Latch15/2
  [VVMC_OVRD2ActRampActive_flg] -> VVMC_OVRD2ActRampActive_flg/1
  Add14/1 -> Divide14/1
  Divide14/1 -> Relational Operator15/2
  Constant73/1 -> Divide14/2
  Divide22/1 -> Relational Operator16/2
  Constant88/1 -> Divide22/2
  [VVMC_ActACCReqAcc4ADS_mps2] -> Min2/2
  Constant96/1 -> Divide24/2
  [VVMC_ActACCRequiredAccel_mps2] -> Divide24/1
  Divide24/1 -> u2 > 0 (1)15/1
  SR_Latch16/1 -> u2 > 0 (1)15/2
  [VVMC_ActACCRequiredAccel_mps2] -> u2 > 0 (1)15/3
  u2 > 0 (1)15/1 -> [VVMC_ActACCReqAcc4ADS_mps2]  "VVMC_ActACCReqAcc4ADS_mps2"
  AND29/1 -> AND19/1
  Detect Increase7/1 -> AND29/1
  [VVMC_ADASWhlTqReachLim_flg] -> Detect Increase7/1
  [VVMC_ReqBrkJoin_flg] -> OR19/3, NOT34/1
  [VVMC_ADASWhlTqReachLim_flg] -> OR20/1
  OR19/1 -> SR_Latch16/1
  NOT34/1 -> SR_Latch16/2
  Constant89/1 -> OR20/2
  OR20/1 -> OR19/1
  Relational Operator82/1 -> SR_Latch14/2
  AND8/1 -> SR_Latch12/1
  [VVMC_ACCVehHoldReqRaw_flg] -> NOT11/1
  NOT11/1 -> SR_Latch12/2
  NOT27/1 -> SR_Latch17/2
  [VVMC_ACCVehHoldReqRaw_flg] -> NOT27/1
  Switch34/1 -> SR_Latch17/1
  Constant29/1 -> OR19/2
  OR16/1 -> OR11/2
  OR21/1 -> OR14/2
